simulink model "LMStry"  (R2015b)
settings: Solver=VariableStepAuto  StartTime=0.0  StopTime=100  RelTol=1e-3
libraries: dspadpt3 x1
settings Model: Creator=User  LastModifiedBy=User

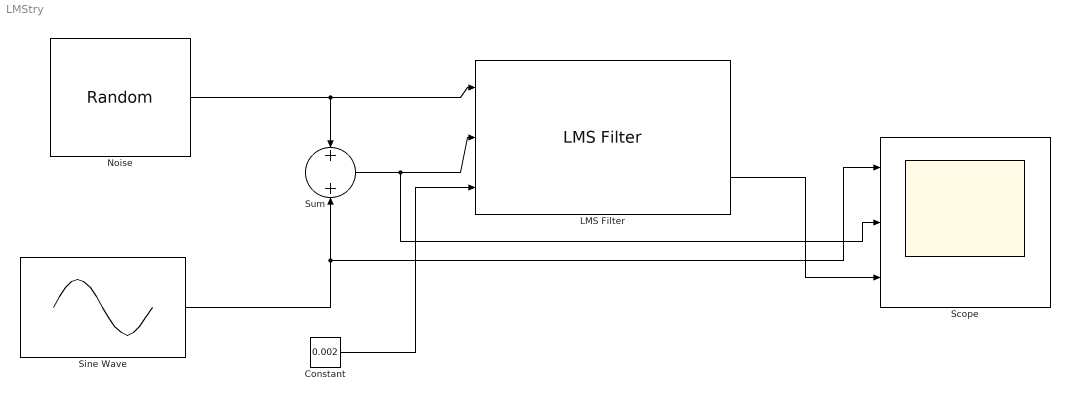
== system LMStry ==
  Constant : Constant  Value=0.002
  LMS Filter : dspadpt3/LMS Filter  Algo=LMS  L=40  stepflag=Input port  mu=0.1  leakage=1.0  ic=0  Adapt=off  resetflag=None  weights=off  secondCoeffMode=User-defined  secondCoeffWordLength=2  secondCoeffFracLength=15  accum2Mode=User-defined  accum2FracLength=20  prodOutput2Mode=User-defined  prodOutput2FracLength=20  prodOutput3Mode=User-defined  prodOutput3FracLength=20  prodOutput4Mode=User-defined  prodOutput4FracLength=20  quotientMode=User-defined  quotientFracLength=20  roundingMode=Floor  overflowMode=off  addnparflag=off
  "Noise " : RandomNumber  Variance=10  SampleTime=0.1
  Scope : Scope  NumInputPorts=3
  Sine Wave : Sin  Frequency=4  SampleTime=0
  Sum : Sum  Inputs=+|+
  wires:
  Sum/1 -> Scope/2, LMS Filter/2
  "Noise "/1 -> Sum/1, LMS Filter/1
  Sine Wave/1 -> Scope/1, Sum/2
  Constant/1 -> LMS Filter/3
  LMS Filter/2 -> Scope/3
